simulink model "HIL_Testing_SW"  (Simulink 7.5)
settings: Solver=ode1  StartTime=0.0  StopTime=Inf  FixedStep=0.001  RelTol=1e-3
PostLoadFcn:
  | , if any(exist('dsrtsu_mdlpostloadfcn', 'file') == [2, 3, 6]), try dsrtsu_mdlpostloadfcn('Execute', bdroot); catch fprintf('Error in PostLoadFcn (dsrtsu_mdlpostloadfcn) for model "%s":\n %s\n', bdroot, lasterr); end, end,
undefined symbols (not defined in the file): CeBSER_Cnt_NumTempAxisPts, ChargeCord, ChargeCord_Control, ChargeToSOCCurr, ChrgCurrLim, CrntSens1Fine, CS_SOCSetPt, CyclerMaxChrgPwr, CyclerMaxDschrgPwr, deltaAhr, Drive_1, Drive_10, Drive_11, Drive_12, Drive_13, Drive_14, Drive_15, Drive_16, Drive_17, Drive_18, Drive_19, Drive_2, Drive_20, Drive_21, Drive_22, Drive_23, Drive_24, Drive_25, Drive_26, Drive_27, Drive_28, Drive_29, Drive_3, Drive_30, Drive_31, Drive_32, Drive_33, Drive_34, Drive_35, Drive_36, Drive_37, Drive_38, Drive_39, Drive_4, Drive_40, Drive_41, Drive_42, Drive_43, Drive_44, Drive_45, Drive_46, Drive_47, Drive_48, Drive_49, Drive_5, Drive_50, Drive_51, Drive_6, Drive_7, Drive_8 ... (+50)
libraries: simulink x129, rtican x50, rti2211sailib x5, rti2211serlib x5, rti2202miolib x3
(part 2 of 23)

== system HIL_Testing_SW/HWO ==
  note: 54A Up is down for DIOs
  ChargeMode : Inport  OutDataType=fixdt(1, 16)  OutScaling=2^0
  PackVoltage : Inport  Port=2  OutDataType=fixdt(1, 16)  OutScaling=2^0
  PackCurrent : Inport  Port=3  OutDataType=fixdt(1, 16)  OutScaling=2^0
  Acc : Constant  Value=0  OutDataTypeMode=boolean  OutDataType=sfix(16)  OutScaling=2^0  OutDataTypeStr=boolean
  AccReset : Constant  Value=0  OutDataTypeMode=boolean  OutDataType=sfix(16)  OutScaling=2^0  OutDataTypeStr=boolean
  Charge : Subsystem
  Compare To Zero1 : simulink/Logic and Bit Operations/Compare To Zero  SystemSampleTime=-1  relop===  LogicOutDataTypeMode=uint8  ZeroCross=off
  Constant : Constant  OutDataType=fixdt(1, 16)  OutScaling=2^0
  ContactorLineActive : Constant  OutDataTypeMode=boolean  OutDataType=fixdt(1, 16)  OutScaling=2^0  OutDataTypeStr=boolean
  DS2202BIT_OUT_B2_C1 : rti2202miolib/DS2202BIT_OUT_B1_C1  SystemSampleTime=-1  DSProperties=struct('RTI',struct('Version',uint32(1),'BlockType',struct('isSLSource',uint8(0),'isSLSink',uint8(1),'isHWSource',uint8(0),'isHWSink',uint8(1),'isSetup',uint8(0),'isInline',uint8(1),'isNonInline',uint8(0),'isInterrupt',uint8(0),'isChannelwise',uint8(1)),'IOBoardType',{{'DS2202','MIO'}},'UnitType','BIT','Identifier','BITOUTCH','DialogType','ML','BlockSet','NONE','SlaveProcessor','NONE'))  RTIBlockInterface=struct('InputPortsWidth',int32(1),'InputPortsActive',1,'InputPortsDataType',{{'SS_BOOLEAN'}},'InputPortsName',{{'BITCH_in'}},'BlockDisplay',{{['BIT OUT\n Channelwise'],'center'}},'IconTransparency','off','InitLevel',2,'DialogFcn','gui2202bitoutch','BlockName',struct('Token',{{'DS2202BIT_OUT_B','_C'}},'BlockParam',{{'BoardNo','ChannelNo'}}),'MaskDescription',['Provides bit-wise write access to the digital output.'],'AddBlockVar',{{'Reserved1','edit','[]';'Reserved2','edit','[]';'Reserved3','edit','[]';'Reserved4','edit','[]'}})  RTIBlockParameters=struct('BoardNo',{{2,'ON',[1 16]}},'ChannelNo',{{1,'ON',[1 16]}},'StateInitValue',{{0,'OFF',[0 1]}},'StateTermMode',{{0,'OFF',[0 1]}},'StateTermValue',{{0,'OFF',[0 1]}},'TLCFileName',{{'rti2202outch','OFF',[]}})  RTISFcnParameters=struct('BoardNo','int32','ChannelNo','int32','StateInitValue','int32','StateTermMode','int32','StateTermValue','int32','TLCFileName','char')  RTIBlockParaDefault=struct('BoardNo',1,'ChannelNo',1,'StateInitValue',0,'StateTermMode',0,'StateTermValue',0,'TLCFileName','rti2202outch')
  DS2202BIT_OUT_B2_C2 : rti2202miolib/DS2202BIT_OUT_B1_C1  SystemSampleTime=-1  DSProperties=struct('RTI',struct('Version',uint32(1),'BlockType',struct('isSLSource',uint8(0),'isSLSink',uint8(1),'isHWSource',uint8(0),'isHWSink',uint8(1),'isSetup',uint8(0),'isInline',uint8(1),'isNonInline',uint8(0),'isInterrupt',uint8(0),'isChannelwise',uint8(1)),'IOBoardType',{{'DS2202','MIO'}},'UnitType','BIT','Identifier','BITOUTCH','DialogType','ML','BlockSet','NONE','SlaveProcessor','NONE'))  RTIBlockInterface=struct('InputPortsWidth',int32(1),'InputPortsActive',1,'InputPortsDataType',{{'SS_BOOLEAN'}},'InputPortsName',{{'BITCH_in'}},'BlockDisplay',{{['BIT OUT\n Channelwise'],'center'}},'IconTransparency','off','InitLevel',2,'DialogFcn','gui2202bitoutch','BlockName',struct('Token',{{'DS2202BIT_OUT_B','_C'}},'BlockParam',{{'BoardNo','ChannelNo'}}),'MaskDescription',['Provides bit-wise write access to the digital output.'],'AddBlockVar',{{'Reserved1','edit','[]';'Reserved2','edit','[]';'Reserved3','edit','[]';'Reserved4','edit','[]'}})  RTIBlockParameters=struct('BoardNo',{{2,'ON',[1 16]}},'ChannelNo',{{2,'ON',[1 16]}},'StateInitValue',{{0,'OFF',[0 1]}},'StateTermMode',{{0,'OFF',[0 1]}},'StateTermValue',{{0,'OFF',[0 1]}},'TLCFileName',{{'rti2202outch','OFF',[]}})  RTISFcnParameters=struct('BoardNo','int32','ChannelNo','int32','StateInitValue','int32','StateTermMode','int32','StateTermValue','int32','TLCFileName','char')  RTIBlockParaDefault=struct('BoardNo',1,'ChannelNo',1,'StateInitValue',0,'StateTermMode',0,'StateTermValue',0,'TLCFileName','rti2202outch')
  DS2211BIT_OUT_B2_C10 : rti2211sailib/DS2211BIT_OUT_B1_C1  SystemSampleTime=-1  DSProperties=struct('RTI',struct('Version',uint32(1),'BlockType',struct('isSLSource',uint8(0),'isSLSink',uint8(1),'isHWSource',uint8(0),'isHWSink',uint8(1),'isSetup',uint8(0),'isInline',uint8(1),'isNonInline',uint8(0),'isInterrupt',uint8(0),'isChannelwise',uint8(1)),'IOBoardType',{{'DS2211','SAI'}},'UnitType','BIT','Identifier','BITOUTCH','DialogType','ML','BlockSet','NONE','SlaveProcessor','NONE'))  RTIBlockInterface=struct('InputPortsWidth',int32(1),'InputPortsActive',1,'InputPortsDataType',{{'SS_BOOLEAN'}},'InputPortsName',{{'BITCH_in'}},'BlockDisplay',{{['BIT OUT\n Channelwise'],'center'}},'IconTransparency','off','InitLevel',2,'DialogFcn','gui2211bitoutch','BlockName',struct('Token',{{'DS2211BIT_OUT_B','_C'}},'BlockParam',{{'BoardNo','ChannelNo'}}),'MaskDescription',['Provides bit-wise write access to the digital output.'],'AddBlockVar',{{'Reserved1','edit','[]';'Reserved2','edit','[]';'Reserved3','edit','[]';'Reserved4','edit','[]'}})  RTIBlockParameters=struct('BoardNo',{{2,'ON',[1 16]}},'ChannelNo',{{10,'ON',[1 16]}},'StateInitValue',{{0,'OFF',[0 1]}},'StateTermMode',{{0,'OFF',[0 1]}},'StateTermValue',{{0,'OFF',[0 1]}},'TLCFileName',{{'rti2211outch','OFF',[]}})  RTISFcnParameters=struct('BoardNo','int32','ChannelNo','int32','StateInitValue','int32','StateTermMode','int32','StateTermValue','int32','TLCFileName','char')  RTIBlockParaDefault=struct('BoardNo',1,'ChannelNo',1,'StateInitValue',0,'StateTermMode',0,'StateTermValue',0,'TLCFileName','rti2211outch')
  DS2211BIT_OUT_B2_C5 : rti2211sailib/DS2211BIT_OUT_B1_C1  SystemSampleTime=-1  DSProperties=struct('RTI',struct('Version',uint32(1),'BlockType',struct('isSLSource',uint8(0),'isSLSink',uint8(1),'isHWSource',uint8(0),'isHWSink',uint8(1),'isSetup',uint8(0),'isInline',uint8(1),'isNonInline',uint8(0),'isInterrupt',uint8(0),'isChannelwise',uint8(1)),'IOBoardType',{{'DS2211','SAI'}},'UnitType','BIT','Identifier','BITOUTCH','DialogType','ML','BlockSet','NONE','SlaveProcessor','NONE'))  RTIBlockInterface=struct('InputPortsWidth',int32(1),'InputPortsActive',1,'InputPortsDataType',{{'SS_BOOLEAN'}},'InputPortsName',{{'BITCH_in'}},'BlockDisplay',{{['BIT OUT\n Channelwise'],'center'}},'IconTransparency','off','InitLevel',2,'DialogFcn','gui2211bitoutch','BlockName',struct('Token',{{'DS2211BIT_OUT_B','_C'}},'BlockParam',{{'BoardNo','ChannelNo'}}),'MaskDescription',['Provides bit-wise write access to the digital output.'],'AddBlockVar',{{'Reserved1','edit','[]';'Reserved2','edit','[]';'Reserved3','edit','[]';'Reserved4','edit','[]'}})  RTIBlockParameters=struct('BoardNo',{{2,'ON',[1 16]}},'ChannelNo',{{5,'ON',[1 16]}},'StateInitValue',{{0,'OFF',[0 1]}},'StateTermMode',{{0,'OFF',[0 1]}},'StateTermValue',{{0,'OFF',[0 1]}},'TLCFileName',{{'rti2211outch','OFF',[]}})  RTISFcnParameters=struct('BoardNo','int32','ChannelNo','int32','StateInitValue','int32','StateTermMode','int32','StateTermValue','int32','TLCFileName','char')  RTIBlockParaDefault=struct('BoardNo',1,'ChannelNo',1,'StateInitValue',0,'StateTermMode',0,'StateTermValue',0,'TLCFileName','rti2211outch')
  DS2211PWM_B2_C7 : rti2211sailib/DS2211PWM_B1_C1  SystemSampleTime=-1  Reserved1=[]  Reserved2=[]  Reserved3=[]  Reserved4=[]  DSProperties=struct('RTI',struct('Version',uint32(1),'BlockType',struct('isSLSource',uint8(0),'isSLSink',uint8(1),'isHWSource',uint8(0),'isHWSink',uint8(1),'isSetup',uint8(0),'isInline',uint8(1),'isNonInline',uint8(0),'isInterrupt',uint8(0),'isChannelwise',uint8(1)),'IOBoardType',{{'DS2211','SAI'}},'UnitType','PWM','Identifier','PWM','DialogType','ML','BlockSet','NONE','SlaveProcessor','NONE'))  RTIBlockInterface=struct('InputPortsWidth',int32([1 1]),'InputPortsActive',[1 1],'InputPortsName',{{['Duty Cycle'],'Period'}},'IconTransparency','on','InitLevel',2,'DialogFcn','gui2211pwm','BlockName',struct('Token',{{'DS2211PWM_B','_C'}},'BlockParam',{{'BoardNo','ChannelNo'}}),'MaskDescription',['Generation of a square-wave-type signal for a given period and duty cycle.'])  RTIBlockParameters=struct('BoardNo',{{2,'ON',[1 16]}},'ChannelNo',{{7,'ON',[1 9]}},'UpdateMode',{{1,'ON',[1 2]}},'PeriodRange',{{2,'OFF',[1 16]}},'DutyCycleInitValue',{{'0.2','OFF',[0 1]}},'PeriodInitValue',{{'1e-005','OFF',[]}},'DutyCyclePeriodTermMode',{{0,'OFF',[0 1]}},'DutyCycleTermValue',{{'0','OFF',[0 1]}},'PeriodTermValue',{{'5e-005','OFF',[]}},'TLCFileName',{{'rti2211pwm','OFF',[]}})  RTISFcnParameters=struct('BoardNo','int32','ChannelNo','int32','UpdateMode','int32','PeriodRange','int32','DutyCycleInitValue','double','PeriodInitValue','double','DutyCyclePeriodTermMode','int32','DutyCycleTermValue','double','PeriodTermValue','double','TLCFileName','char')  RTIBlockParaDefault=struct('BoardNo',1,'ChannelNo',1,'UpdateMode',1,'PeriodRange',7,'DutyCycleInitValue',0,'PeriodInitValue',5e-05,'DutyCyclePeriodTermMode',0,'DutyCycleTermValue',0,'PeriodTermValue',5e-05,'TLCFileName','rti2211pwm')
  DS2211PWM_B2_C9 : rti2211sailib/DS2211PWM_B1_C1  SystemSampleTime=-1  Reserved1=[]  Reserved2=[]  Reserved3=[]  Reserved4=[]  DSProperties=struct('RTI',struct('Version',uint32(1),'BlockType',struct('isSLSource',uint8(0),'isSLSink',uint8(1),'isHWSource',uint8(0),'isHWSink',uint8(1),'isSetup',uint8(0),'isInline',uint8(1),'isNonInline',uint8(0),'isInterrupt',uint8(0),'isChannelwise',uint8(1)),'IOBoardType',{{'DS2211','SAI'}},'UnitType','PWM','Identifier','PWM','DialogType','ML','BlockSet','NONE','SlaveProcessor','NONE'))  RTIBlockInterface=struct('InputPortsWidth',int32([1 1]),'InputPortsActive',[1 1],'InputPortsName',{{['Duty Cycle'],'Period'}},'IconTransparency','on','InitLevel',2,'DialogFcn','gui2211pwm','BlockName',struct('Token',{{'DS2211PWM_B','_C'}},'BlockParam',{{'BoardNo','ChannelNo'}}),'MaskDescription',['Generation of a square-wave-type signal for a given period and duty cycle.'])  RTIBlockParameters=struct('BoardNo',{{2,'ON',[1 16]}},'ChannelNo',{{9,'ON',[1 9]}},'UpdateMode',{{1,'ON',[1 2]}},'PeriodRange',{{3,'OFF',[1 16]}},'DutyCycleInitValue',{{'0.2','OFF',[0 1]}},'PeriodInitValue',{{'1e-005','OFF',[]}},'DutyCyclePeriodTermMode',{{0,'OFF',[0 1]}},'DutyCycleTermValue',{{'0','OFF',[0 1]}},'PeriodTermValue',{{'5e-005','OFF',[]}},'TLCFileName',{{'rti2211pwm','OFF',[]}})  RTISFcnParameters=struct('BoardNo','int32','ChannelNo','int32','UpdateMode','int32','PeriodRange','int32','DutyCycleInitValue','double','PeriodInitValue','double','DutyCyclePeriodTermMode','int32','DutyCycleTermValue','double','PeriodTermValue','double','TLCFileName','char')  RTIBlockParaDefault=struct('BoardNo',1,'ChannelNo',1,'UpdateMode',1,'PeriodRange',7,'DutyCycleInitValue',0,'PeriodInitValue',5e-05,'DutyCyclePeriodTermMode',0,'DutyCycleTermValue',0,'PeriodTermValue',5e-05,'TLCFileName','rti2211pwm')
  Data Store Read : DataStoreRead  DataStoreName=fault  SampleTime=0
  Data Store Read1 : DataStoreRead  DataStoreName=ResetRun  SampleTime=0
  Data Store Read2 : DataStoreRead  DataStoreName=ResetRun  SampleTime=0
  Data Store Write : DataStoreWrite  DataStoreName=ContactorLine  SampleTime=-1
  Data Store Write1 : DataStoreWrite  DataStoreName=ACC  SampleTime=-1
  Data Store Write2 : DataStoreWrite  DataStoreName=RUN  SampleTime=-1
  Divide : Product  Inputs=*/  OutDataType=fixdt(1, 16)  OutScaling=2^-10
  DriveSelect4 : Switch  Threshold=0.5  OutDataType=fixdt(1, 16)  OutScaling=2^0
  DriveSelect6 : Switch  Threshold=0.5  OutDataType=fixdt(1, 16)  OutScaling=2^0
  Logical Operator : Logic  Operator=NOT  AllPortsSameDT=off  OutDataTypeMode=boolean  LogicDataType=fixdt(0, 8)  OutDataTypeStr=boolean
  Logical Operator3 : Logic  AllPortsSameDT=off  OutDataTypeMode=boolean  LogicDataType=fixdt(0, 8)  OutDataTypeStr=boolean
  Logical Operator8 : Logic  Operator=OR  AllPortsSameDT=off  OutDataTypeMode=boolean  LogicDataType=fixdt(0, 8)  OutDataTypeStr=boolean
  Reset_Run : Constant  Value=0  OutDataTypeMode=boolean  OutDataType=fixdt(1, 16)  OutScaling=2^0  OutDataTypeStr=boolean
  Run : Constant  Value=0  OutDataTypeMode=boolean  OutDataType=fixdt(1, 16)  OutScaling=2^0  OutDataTypeStr=boolean
  Switch1 : Switch  Threshold=.5  OutDataType=fixdt(1, 16)  OutScaling=2^0
  TX HVEM : Subsystem
  Ignition : Outport  OutDataType=fixdt(1, 16)  OutScaling=2^0
  tag scope: ChargeMode=global, Ignition=global, PackCurrent=global, PackVoltage=global
  wires:
  [DC] -> DS2211PWM_B2_C7/1
  [Period] -> DS2211PWM_B2_C7/2
  [Prox] -> DS2211BIT_OUT_B2_C5/1
  AccReset/1 -> DriveSelect6/1
  Data Store Read2/1 -> DriveSelect6/2
  DriveSelect6/1 -> Data Store Write1/1, DS2202BIT_OUT_B2_C1/1
  DriveSelect4/1 -> DS2211BIT_OUT_B2_C10/1, Data Store Write/1
  ContactorLineActive/1 -> DriveSelect4/1
  [ChargeMode] -> DriveSelect4/2
  [Ignition] -> Logical Operator3/1
  Data Store Read/1 -> Compare To Zero1/1
  Compare To Zero1/1 -> Logical Operator3/2
  Logical Operator3/1 -> DriveSelect4/3
  Acc/1 -> DriveSelect6/3
  Switch1/1 -> Ignition/1, Data Store Write2/1, [Ignition], DS2202BIT_OUT_B2_C2/1
  Reset_Run/1 -> Switch1/1
  Run/1 -> Switch1/3
  Logical Operator8/1 -> Switch1/2
  Data Store Read1/1 -> Logical Operator8/1
  ChargeMode/1 -> [ChargeMode]
  [ChargeMode] -> Logical Operator8/2
  Logical Operator/1 -> Charge/Enable
  [ChargeMode] -> Logical Operator/1
  Charge/1(Period_1) -> [Period1]
  Charge/2(DC1) -> [DC1]
  Charge/3(Prox) -> [Prox1]
  TX HVEM/1(DC) -> [DC]
  TX HVEM/2(Period) -> [Period]
  TX HVEM/3(Proximity) -> [Prox]
  [PackCurrent] -> TX HVEM/1(Current)
  [ChargeMode] -> TX HVEM/2(CM)
  [PackVoltage] -> TX HVEM/3(Voltage)
  PackVoltage/1 -> [PackVoltage]
  PackCurrent/1 -> [PackCurrent]
  TX HVEM/4(PrcsdVolt_DC) -> [PrcsdVolt_DC]
  TX HVEM/5(PrcsdVolt_Period) -> [PrcsdVolt_Freq]
  [PrcsdVolt_Freq] -> DS2211PWM_B2_C9/2
  Constant/1 -> Divide/2
  [PrcsdVolt_DC] -> Divide/1
  Divide/1 -> DS2211PWM_B2_C9/1

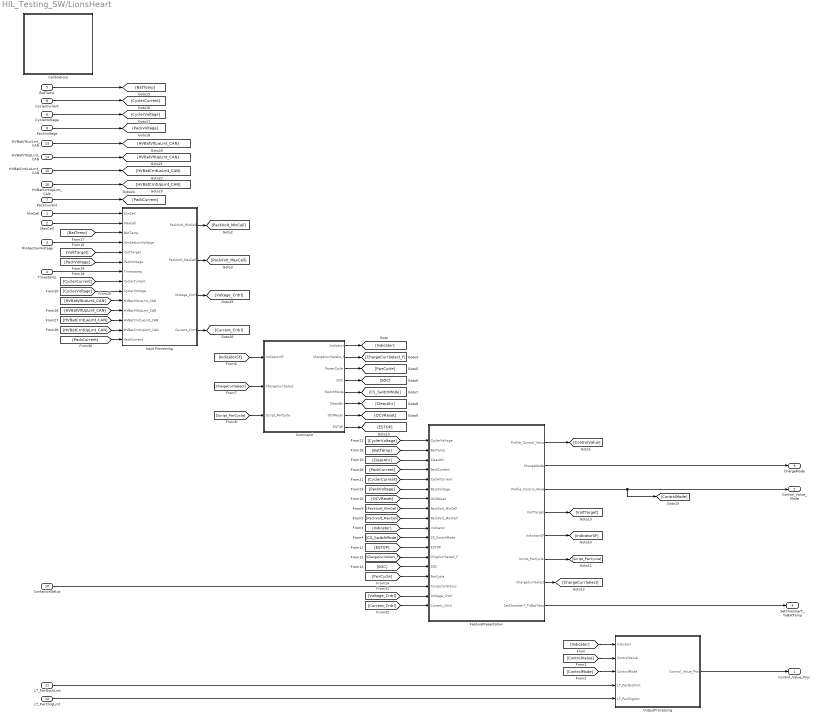
== system HIL_Testing_SW/LionsHeart ==
  MinCell : Inport  OutDataType=fixdt(1, 16)  OutScaling=2^0
  MaxCell : Inport  Port=2  OutDataType=fixdt(1, 16)  OutScaling=2^0
  MinSectionVoltage : Inport  Port=3  OutDataType=fixdt(1, 16)  OutScaling=2^0
  Timestamp : Inport  Port=4  OutDataType=fixdt(1, 16)  OutScaling=2^0
  BatTemp : Inport  Port=5  OutDataType=fixdt(1, 16)  OutScaling=2^0
  CyclerVoltage : Inport  Port=6  OutDataType=fixdt(1, 16)  OutScaling=2^0
  PackCurrent : Inport  Port=7  OutDataType=fixdt(1, 16)  OutScaling=2^0
  CyclerCurrent : Inport  Port=8  OutDataType=fixdt(1, 16)  OutScaling=2^0
  PackVoltage : Inport  Port=9  OutDataType=fixdt(1, 16)  OutScaling=2^0
  ContactorStatus : Inport  Port=10  OutDataType=fixdt(1, 16)  OutScaling=2^0
  LT_PwrDschLmt : Inport  Port=11  OutDataType=fixdt(1, 16)  OutScaling=2^0
  LT_PwrChrgLmt : Inport  Port=12  OutDataType=fixdt(1, 16)  OutScaling=2^0
  HVBatVltLwLmt_CAN : Inport  Port=13  OutDataType=fixdt(1, 16)  OutScaling=2^0
  HVBatVltUpLmt_CAN : Inport  Port=14  OutDataType=fixdt(1, 16)  OutScaling=2^0
  HVBatCrntLwLmt_CAN : Inport  Port=15  OutDataType=fixdt(1, 16)  OutScaling=2^0
  HVBatCrntUpLmt_CAN : Inport  Port=16  OutDataType=fixdt(1, 16)  OutScaling=2^0
  Calibrations : Subsystem
  Command : Subsystem
  FeaturePresentation : Subsystem
  Input Processing : Subsystem
  OutputProcessing : Subsystem
  Control_Value_Proc : Outport  OutDataType=fixdt(1, 16)  OutScaling=2^0
  Control_Value_Mode : Outport  Port=2  OutDataType=fixdt(1, 16)  OutScaling=2^0
  ChargeMode : Outport  Port=3  OutDataType=fixdt(1, 16)  OutScaling=2^0
  SetChamberT_ToBatTemp : Outport  Port=4  OutDataType=fixdt(1, 16)  OutScaling=2^0
  wires:
  OutputProcessing/1(Control_Value_Proc) -> Control_Value_Proc/1
  LT_PwrDschLmt/1 -> OutputProcessing/4(LT_PwrDschlmt)
  LT_PwrChrgLmt/1 -> OutputProcessing/5(LT_PwrChgLmt)
  Command/1(Indicator) -> [Indicator]
  [Indicator] -> OutputProcessing/1(Indicator)
  FeaturePresentation/1(Profile_Control_Value) -> [ControlValue]
  FeaturePresentation/3(Profile_Control_Mode) -> Control_Value_Mode/1, [ControlMode]
  [ControlValue] -> OutputProcessing/2(ControlValue)
  [ControlMode] -> OutputProcessing/3(ControlMode)
  [Indicator] -> FeaturePresentation/10(Indicator)
  Input Processing/1(PackVolt_MinCell) -> [PackVolt_MinCell]
  Input Processing/2(PackVolt_MaxCell) -> [PackVolt_MaxCell]
  FeaturePresentation/2(ChargeMode) -> ChargeMode/1
  [CS_SwitchMode] -> FeaturePresentation/11(CS_SwitchMode)
  [PackVolt_MaxCell] -> FeaturePresentation/9(PackVolt_MaxCell)
  Command/2(ChargeCurrSelect_F) -> [ChargeCurrSelect_F]
  Command/3(PowerCycle) -> [PwrCycle]
  Command/4(SOC) -> [SOC]
  Command/5(SwitchMode) -> [CS_SwitchMode]
  Command/6(ClearAhr) -> [ClearAhr]
  Command/7(OCVReset) -> [OCVReset]
  [IndicatorSF] -> Command/1(IndicatorSF)
  [ChargeCurrSelect] -> Command/2(ChargeCurrSelect)
  FeaturePresentation/5(IndicatorSF) -> [IndicatorSF]
  FeaturePresentation/6(Script_PwrCycle) -> [Script_PwrCycle]
  FeaturePresentation/7(ChargeCurrSelect) -> [ChargeCurrSelect]
  FeaturePresentation/4(VoltTarget) -> [VoltTarget]
  [Script_PwrCycle] -> Command/3(Script_PwrCycle)
  [PackVolt_MinCell] -> FeaturePresentation/8(PackVolt_MinCell)
  [OCVReset] -> FeaturePresentation/7(OCVReset)
  Command/8(ESTOP) -> [ESTOP]
  [ESTOP] -> FeaturePresentation/12(ESTOP)
  [ChargeCurrSelect_F] -> FeaturePresentation/13(ChrgCurrSelect_F)
  [SOC] -> FeaturePresentation/14(SOC)
  [PwrCycle] -> FeaturePresentation/15(PwrCycle)
  [ClearAhr] -> FeaturePresentation/3(ClearAhr)
  [VoltTarget] -> Input Processing/5(VoltTarget)
  MinCell/1 -> Input Processing/1(MinCell)
  MaxCell/1 -> Input Processing/2(MaxCell)
  MinSectionVoltage/1 -> Input Processing/4(MinSectionVoltage)
  Timestamp/1 -> Input Processing/7(Timestamp)
  BatTemp/1 -> [BatTemp]
  [BatTemp] -> Input Processing/3(BatTemp)
  [BatTemp] -> FeaturePresentation/2(BatTemp)
  ContactorStatus/1 -> FeaturePresentation/16(ContactorStatus)
  CyclerCurrent/1 -> [CyclerCurrent]
  CyclerVoltage/1 -> [CyclerVoltage]
  [CyclerCurrent] -> Input Processing/8(CyclerCurrent)
  [CyclerVoltage] -> Input Processing/9(CyclerVotlage)
  [CyclerCurrent] -> FeaturePresentation/5(CyclerCurrent)
  [CyclerVoltage] -> FeaturePresentation/1(CyclerVoltage)
  [PackVoltage] -> FeaturePresentation/6(PackVoltage)
  PackVoltage/1 -> [PackVoltage]
  [PackVoltage] -> Input Processing/6(PackVoltage)
  HVBatVltLwLmt_CAN/1 -> [HVBatVltLwLmt_CAN]
  HVBatVltUpLmt_CAN/1 -> [HVBatVltUpLmt_CAN]
  HVBatCrntLwLmt_CAN/1 -> [HVBatCrntLwLmt_CAN]
  HVBatCrntUpLmt_CAN/1 -> [HVBatCrntUpLmt_CAN]
  [HVBatVltLwLmt_CAN] -> Input Processing/10(HVBatVltLwLmt_CAN)
  [HVBatVltUpLmt_CAN] -> Input Processing/11(HVBatVltUpLmt_CAN)
  [HVBatCrntLwLmt_CAN] -> Input Processing/12(HVBatCrntLwLmt_CAN)
  [HVBatCrntUpLmt_CAN] -> Input Processing/13(HVBatCrntUpLmt_CAN)
  PackCurrent/1 -> [PackCurrent]
  [PackCurrent] -> FeaturePresentation/4(PackCurrent)
  [PackCurrent] -> Input Processing/14(PackCurrent)
  Input Processing/3(Voltage_Cntrl) -> [Voltage_Cntrl]
  Input Processing/4(Current_Cntrl) -> [Current_Cntrl]
  [Voltage_Cntrl] -> FeaturePresentation/17(Voltage_Cntrl)
  [Current_Cntrl] -> FeaturePresentation/18(Current_Cntrl)
  FeaturePresentation/8(SetChamberT_ToBatTemp) -> SetChamberT_ToBatTemp/1

== system HIL_Testing_SW/RTI Data ==
  RTI Data Store : Subsystem  Tag="struct('private',struct('version',struct('dsVer',uint32(2),'dsVerCreation',uint32(2),'RTI',struct('ver','6.7','type','RTI1006')),'access',struct('type','Model','isPerm',1,'created',['10-Dec-2012 12:09:16'],'modified',['22-Sep-2015 13:45:03'],'location','')),'public',struct('main',struct('data',[]),'sub',struct('name',{{'HIL_Testing_SW'}},'data',{{struct('TH',struct('thTaskInfo',struct('taskType',{'TIMER','HWINT','TMRINT','SWINT'},'tasksNumOf',{7,0,0,0},'srcIds',{{'TIMERA','TIMERA2','TIMERA3','TIMERA4','TIMERA5','TIMERA6','TIMERA7'},{},{},{}},'taskNames',{{['Timer Task 1'],['Timer Task 2'],['Timer Task 3'],['Timer Task 4'],['Timer Task 5'],['Timer Task 6'],['Timer Task 7']},{},{},{}})),'th_tc',struct('dataType',{'TASK','TASK','TASK','TASK','TASK','TASK','TASK'},'taskGroupId',{'','','','','','',''},'taskGroupList',{{},{},{},{},{},{},{}},'taskSchedulingPolicy',{'FCFS','FCFS','FCFS','FCFS','FCFS','FCFS','FCFS'},'taskType',{'TIMER','TIMER','TIMER','TIMER','TIMER','TIMER','TIMER'},'blkh',{-1,-1,-1,-1,-1,-1,-1},'srcId',{'TIMERA','TIMERA2','TIMERA3','TIMERA4','TIMERA5','TIMERA6','TIMERA7'},'srcSgnName',{['Timer A interrupt'],['Timer Task 1'],['Timer Task 1'],['Timer Task 1'],['Timer Task 1'],['Timer Task 1'],['Timer Task 1']},'srcCpuName',{'','','','','','',''},'taskName',{['Timer Task 1  [0.001] s'],['Timer Task 2  [0.012] s'],['Timer Task 3  [0.025] s'],['Timer Task 4  [0.2] s'],['Timer Task 5  [0.3] s'],['Timer Task 6  [0.4] s'],['Timer Task 7  [1] s']},'taskNameDisplayExt',{'','','','','','',''},'smplTime',{0.001,0.012,0.025,0.2,0.3,0.4,1},'smplTimeOffs',{0,0,0,0,0,0,0},'hasFixedPriority',{0,0,0,0,0,0,0},'priority',{1,2,3,4,5,6,7},'hasFixedOvc',{0,0,0,0,0,0,0},'ovcType',{1,1,1,1,1,1,1},'ovcMax',{1,1,1,1,1,1,1}),'tc_th',struct('dataType',{'TASK','TASK','TASK','TASK','TASK','TASK','TASK'},'taskGroupId',{'','','','','','',''},'taskGroupList',{{},{},{},{},{},{},{}},'taskSchedulingPolicy',{'FCFS','FCFS','FCFS','FCFS','FCFS','FCFS','FCFS'},'taskType',{'TIMER','TIMER','TIMER','TIMER','TIMER','TIMER','TIMER'},'blkh',{-1,-1,-1,-1,-1,-1,-1},'srcId',{'TIMERA','TIMERA2','TIMERA3','TIMERA4','TIMERA5','TIMERA6','TIMERA7'},'srcSgnName',{['Timer A interrupt'],['Timer Task 1'],['Timer Task 1'],['Timer Task 1'],['Timer Task 1'],['Timer Task 1'],['Timer Task 1']},'srcCpuName',{'','','','','','',''},'taskName',{['Timer Task 1  [0.001] s'],['Timer Task 2  [0.012] s'],['Timer Task 3  [0.025] s'],['Timer Task 4  [0.2] s'],['Timer Task 5  [0.3] s'],['Timer Task 6  [0.4] s'],['Timer Task 7  [1] s']},'taskNameDisplayExt',{'','','','','','',''},'smplTime',{0.001,0.012,0.025,0.2,0.3,0.4,1},'smplTimeOffs',{0,0,0,0,0,0,0},'hasFixedPriority',{0,0,0,0,0,0,0},'priority',{1,2,3,4,5,6,7},'hasFixedOvc',{0,0,0,0,0,0,0},'ovcType',{1,1,1,1,1,1,1},'ovcMax',{1,1,1,1,1,1,1}))}})))"
      mask Type: RTI_DATA_STORE
      mask Description:
      | RTI Data Store Block. This block is used by RTI to store internal model dependent data. Deleting this block will result in data loss.
      | 
      | NEVER DELETE, COPY, OR MODIFY THIS BLOCK!
      mask Help:
      | RTI Data Store Block. This block is used by RTI to store internal model dependent data. Deleting this block will result in data loss.
      | 
      | NEVER DELETE, COPY, OR MODIFY THIS BLOCK!
      mask Display: text(0.5, 0.5, ' ', 'HorizontalAlignment', 'center');

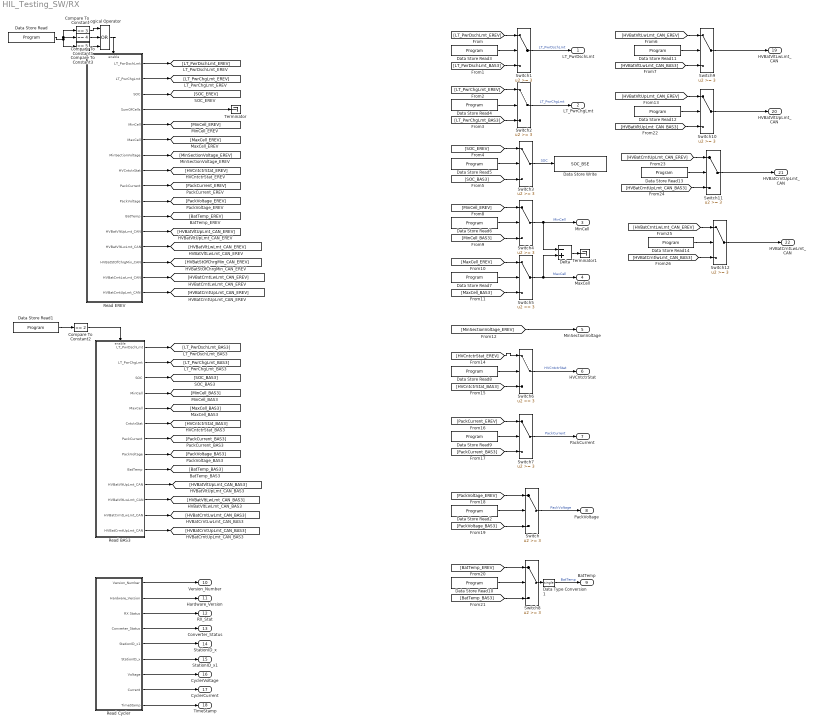
== system HIL_Testing_SW/RX ==
  Compare To Constant : simulink/Logic and Bit Operations/Compare To Constant  SystemSampleTime=-1  relop===  const=3  LogicOutDataTypeMode=uint8
  Compare To Constant1 : simulink/Logic and Bit Operations/Compare To Constant  SystemSampleTime=-1  relop===  const=4  LogicOutDataTypeMode=uint8
  Compare To Constant2 : simulink/Logic and Bit Operations/Compare To Constant  SystemSampleTime=-1  relop===  const=2  LogicOutDataTypeMode=uint8
  Compare To Constant3 : simulink/Logic and Bit Operations/Compare To Constant  SystemSampleTime=-1  relop===  const=5  LogicOutDataTypeMode=uint8
  Data Store Read{,1..14} (15 alike) : DataStoreRead  DataStoreName=Program  SampleTime=0
  Data Store Write : DataStoreWrite  DataStoreName=SOC_BSE  SampleTime=-1
  Data Type Conversion1 : DataTypeConversion  OutDataTypeMode=single  OutDataType=fixdt(1, 16)  OutScaling=2^0  OutDataTypeStr=single
  Delta : Sum  Inputs=-+  OutDataType=fixdt(1, 16)  OutScaling=2^-10
  Logical Operator : Logic  Operator=OR  Inputs=3  AllPortsSameDT=off  OutDataTypeMode=boolean  LogicDataType=fixdt(0, 8)  OutDataTypeStr=boolean
  Read BAS3 : Subsystem
  Read Cycler : Subsystem
  Read EREV : Subsystem
  Switch{,1..12} (13 alike) : Switch  Threshold=3  OutDataType=sfix(16)  OutScaling=2^0
  Terminator : Terminator
  Terminator1 : Terminator
  LT_PwrDschLmt : Outport  OutDataType=fixdt(1, 16)  OutScaling=2^0
  LT_PwrChgLmt : Outport  Port=2  OutDataType=fixdt(1, 16)  OutScaling=2^0
  MinCell : Outport  Port=3  OutDataType=fixdt(1, 16)  OutScaling=2^0
  MaxCell : Outport  Port=4  OutDataType=fixdt(1, 16)  OutScaling=2^0
  MinSectionVoltage : Outport  Port=5  OutDataType=fixdt(1, 16)  OutScaling=2^0
  HVCntctrStat : Outport  Port=6  OutDataType=fixdt(1, 16)  OutScaling=2^0
  PackCurrent : Outport  Port=7  OutDataType=fixdt(1, 16)  OutScaling=2^0
  PackVoltage : Outport  Port=8  OutDataType=fixdt(1, 16)  OutScaling=2^0
  BatTemp : Outport  Port=9  OutDataType=fixdt(1, 16)  OutScaling=2^0
  Version_Number : Outport  Port=10  OutDataType=fixdt(1, 16)  OutScaling=2^0
  Hardware_Version : Outport  Port=11  OutDataType=fixdt(1, 16)  OutScaling=2^0
  RX_Stat : Outport  Port=12  OutDataType=fixdt(1, 16)  OutScaling=2^0
  Converter_Status : Outport  Port=13  OutDataType=fixdt(1, 16)  OutScaling=2^0
  StationID_x : Outport  Port=14  OutDataType=fixdt(1, 16)  OutScaling=2^0
  StationID_x1 : Outport  Port=15  OutDataType=fixdt(1, 16)  OutScaling=2^0
  CyclerVoltage : Outport  Port=16  OutDataType=fixdt(1, 16)  OutScaling=2^0
  CyclerCurrent : Outport  Port=17  OutDataType=fixdt(1, 16)  OutScaling=2^0
  TimeStamp : Outport  Port=18  OutDataType=fixdt(1, 16)  OutScaling=2^0
  HVBatVltLwLmt_CAN : Outport  Port=19  OutDataType=fixdt(1, 16)  OutScaling=2^0
  HVBatVltUpLmt_CAN : Outport  Port=20  OutDataType=fixdt(1, 16)  OutScaling=2^0
  HVBatCrntUpLmt_CAN : Outport  Port=21  OutDataType=fixdt(1, 16)  OutScaling=2^0
  HVBatCrntLwLmt_CAN : Outport  Port=22  OutDataType=fixdt(1, 16)  OutScaling=2^0
  wires:
  Read EREV/2(LT_PwrChgLmt) -> [LT_PwrChgLmt_EREV]
  Read EREV/1(LT_PwrDschLmt) -> [LT_PwrDschLmt_EREV]
  Read EREV/3(SOC) -> [SOC_EREV]
  Read EREV/4(SumOfCells) -> Terminator/1
  Read EREV/5(MinCell) -> [MinCell_EREV]
  Read EREV/6(MaxCell) -> [MaxCell_EREV]
  Read EREV/7(MinSectionVoltage) -> [MinSectionVoltage_EREV]
  Read EREV/8(HVCntctrStat) -> [HVCntctrStat_EREV]
  Read EREV/9(PackCurrent) -> [PackCurrent_EREV]
  Read EREV/10(PackVoltage) -> [PackVoltage_EREV]
  Read EREV/11(BatTemp) -> [BatTemp_EREV]
  Switch/1 -> PackVoltage/1  "PackVoltage"
  Read BAS3/1(LT_PwrDschLmt) -> [LT_PwrDschLmt_BAS3]
  Read BAS3/2(LT_PwrChgLmt) -> [LT_PwrChgLmt_BAS3]
  Read BAS3/3(SOC) -> [SOC_BAS3]
  Read BAS3/4(MinCell) -> [MinCell_BAS3]
  Read BAS3/5(MaxCell) -> [MaxCell_BAS3]
  Read BAS3/6(CntctrStat) -> [HVCntctrStat_BAS3]
  Read BAS3/7(PackCurrent) -> [PackCurrent_BAS3]
  Read BAS3/8(PackVoltage) -> [PackVoltage_BAS3]
  Read BAS3/9(BatTemp) -> [BatTemp_BAS3]
  [MinSectionVoltage_EREV] -> MinSectionVoltage/1
  Data Store Read/1 -> Compare To Constant/1, Compare To Constant1/1, Compare To Constant3/1
  Compare To Constant/1 -> Logical Operator/1
  Compare To Constant1/1 -> Logical Operator/2
  Logical Operator/1 -> Read EREV/Enable
  Data Store Read1/1 -> Compare To Constant2/1
  Compare To Constant2/1 -> Read BAS3/Enable
  Read Cycler/1(Version_Number) -> Version_Number/1
  Read Cycler/2(Hardware_Version) -> Hardware_Version/1
  Read Cycler/3(RX Status) -> RX_Stat/1
  Read Cycler/4(Converter_Status) -> Converter_Status/1
  Read Cycler/5(StationID_x1) -> StationID_x/1
  Read Cycler/6(StationID_x) -> StationID_x1/1
  Read Cycler/7(Voltage) -> CyclerVoltage/1
  Read Cycler/8(Current) -> CyclerCurrent/1
  Read Cycler/9(TimeStamp) -> TimeStamp/1
  Data Type Conversion1/1 -> BatTemp/1  "BatTemp"
  Data Store Read2/1 -> Switch/2
  [PackVoltage_BAS3] -> Switch/3
  [PackVoltage_EREV] -> Switch/1
  [LT_PwrDschLmt_BAS3] -> Switch1/3
  [LT_PwrDschLmt_EREV] -> Switch1/1
  Data Store Read3/1 -> Switch1/2
  Switch1/1 -> LT_PwrDschLmt/1  "LT_PwrDschLmt"
  Data Store Read4/1 -> Switch2/2
  [LT_PwrChgLmt_EREV] -> Switch2/1
  [LT_PwrChgLmt_BAS3] -> Switch2/3
  Switch2/1 -> LT_PwrChgLmt/1  "LT_PwrChgLmt"
  [SOC_EREV] -> Switch3/1
  [SOC_BAS3] -> Switch3/3
  Data Store Read5/1 -> Switch3/2
  Switch3/1 -> Data Store Write/1  "SOC"
  [MinCell_BAS3] -> Switch4/3
  [MinCell_EREV] -> Switch4/1
  Data Store Read6/1 -> Switch4/2
  Switch4/1 -> MinCell/1, Delta/1  "MinCell"
  [MaxCell_EREV] -> Switch5/1
  [MaxCell_BAS3] -> Switch5/3
  Data Store Read7/1 -> Switch5/2
  Switch5/1 -> MaxCell/1, Delta/2  "MaxCell"
  [HVCntctrStat_EREV] -> Switch6/1
  [HVCntctrStat_BAS3] -> Switch6/3
  Data Store Read8/1 -> Switch6/2
  Switch6/1 -> HVCntctrStat/1  "HVCntctrStat"
  [PackCurrent_EREV] -> Switch7/1
  [PackCurrent_BAS3] -> Switch7/3
  Data Store Read9/1 -> Switch7/2
  Switch7/1 -> PackCurrent/1  "PackCurrent"
  [BatTemp_EREV] -> Switch8/1
  [BatTemp_BAS3] -> Switch8/3
  Data Store Read10/1 -> Switch8/2
  Switch8/1 -> Data Type Conversion1/1
  Read EREV/12(HVBatVltUpLmt_CAN) -> [HVBatVltUpLmt_CAN_EREV]
  Read EREV/13(HVBatVltLwLmt_CAN) -> [HVBatVltLwLmt_CAN_EREV]
  Read EREV/14(HVBatStOfChrgMin_CAN) -> [HVBatStOfChrgMin_CAN_EREV]
  Read EREV/15(HVBatCrntLwLmt_CAN) -> [HVBatCrntLwLmt_CAN_EREV]
  Read EREV/16(HVBatCrntUpLmt_CAN) -> [HVBatCrntUpLmt_CAN_EREV]
  Read BAS3/10(HVBatVltUpLmt_CAN) -> [HVBatVltUpLmt_CAN_BAS3]
  [HVBatVltLwLmt_CAN_BAS3] -> Switch9/3
  [HVBatVltLwLmt_CAN_EREV] -> Switch9/1
  Data Store Read11/1 -> Switch9/2
  Read BAS3/11(HVBatVltLwLmt_CAN) -> [HVBatVltLwLmt_CAN_BAS3]
  Read BAS3/12(HVBatCrmtLwLmt_CAN) -> [HVBatCrntLwLmt_CAN_BAS3]
  Read BAS3/13(HVBatCrmtUpLmt_CAN) -> [HVBatCrntUpLmt_CAN_BAS3]
  Switch9/1 -> HVBatVltLwLmt_CAN/1
  [HVBatVltUpLmt_CAN_BAS3] -> Switch10/3
  [HVBatVltUpLmt_CAN_EREV] -> Switch10/1
  Data Store Read12/1 -> Switch10/2
  Switch10/1 -> HVBatVltUpLmt_CAN/1
  [HVBatCrntUpLmt_CAN_BAS3] -> Switch11/3
  [HVBatCrntUpLmt_CAN_EREV] -> Switch11/1
  Data Store Read13/1 -> Switch11/2
  Switch11/1 -> HVBatCrntUpLmt_CAN/1
  [HVBatCrntlwLmt_CAN_BAS3] -> Switch12/3
  [HVBatCrntLwLmt_CAN_EREV] -> Switch12/1
  Data Store Read14/1 -> Switch12/2
  Switch12/1 -> HVBatCrntLwLmt_CAN/1
  Compare To Constant3/1 -> Logical Operator/3
  Delta/1 -> Terminator1/1

== system HIL_Testing_SW/TX ==
  note: Place holder for future use!
      | SDE 0821
  Version_Number : Inport  OutDataType=sfix(16)  OutScaling=2^0
  Hardware_Version : Inport  Port=2  OutDataType=sfix(16)  OutScaling=2^0
  Rx_status : Inport  Port=3  OutDataType=sfix(16)  OutScaling=2^0
  Converter_Status : Inport  Port=4  OutDataType=sfix(16)  OutScaling=2^0
  StationID_x1 : Inport  Port=5  OutDataType=sfix(16)  OutScaling=2^0
  StationID_x : Inport  Port=6  OutDataType=sfix(16)  OutScaling=2^0
  Control_Value_Proc : Inport  Port=7  OutDataType=sfix(16)  OutScaling=2^0
  Control_Mode : Inport  Port=8  OutDataType=sfix(16)  OutScaling=2^0
  BatTemp : Inport  Port=9  OutDataType=sfix(16)  OutScaling=2^0
  PackVoltage : Inport  Port=10  OutDataType=sfix(16)  OutScaling=2^0
  Ignition : Inport  Port=11  OutDataType=sfix(16)  OutScaling=2^0
  SetChamberT_ToBatTemp : Inport  Port=12  OutDataType=sfix(16)  OutScaling=2^0
  Chamber : Subsystem
  Chiller : Subsystem
  Data Store Read : DataStoreRead  DataStoreName=ContactorLine  SampleTime=0
  Data Store Read1 : DataStoreRead  DataStoreName=ContactorLine  SampleTime=0
  Data Store Read2 : DataStoreRead  DataStoreName=ContactorLine  SampleTime=0
  ProfBatt_Temp : Constant  Value=single(25.1)  OutDataType=fixdt(1, 16)  OutScaling=2^0
  PrpslnAtv : Subsystem
  TX PTEI : Subsystem
  Tx_Cycler : Subsystem
  wires:
  Version_Number/1 -> Tx_Cycler/3(Version_Number)
  Hardware_Version/1 -> Tx_Cycler/4(Hardware_Version)
  Rx_status/1 -> Tx_Cycler/5(Rx_status)
  Converter_Status/1 -> Tx_Cycler/6(Converter_Status_B)
  Data Store Read1/1 -> TX PTEI/3(ContactorLine)
  Data Store Read2/1 -> PrpslnAtv/1(ContactorLine)
  BatTemp/1 -> [Temp]
  PackVoltage/1 -> [PackVoltage]
  Ignition/1 -> [Ignition]
  [PackVoltage] -> TX PTEI/1(BatVolt)
  [Ignition] -> TX PTEI/2(Ignition)
  Control_Value_Proc/1 -> Tx_Cycler/1(Control_Value_Proc)
  Control_Mode/1 -> Tx_Cycler/2(Control_Mode)
  StationID_x1/1 -> Tx_Cycler/7(StationID_B1)
  StationID_x/1 -> Tx_Cycler/8(StationID_B)
  [Temp] -> Chamber/1(BatTemp)
  SetChamberT_ToBatTemp/1 -> [SetChamberT_ToBatTemp]
  [SetChamberT_ToBatTemp] -> Chamber/2(SetChamberT_ToBatTemp)
  [Temp] -> Chiller/1(BatTemp)
  Data Store Read/1 -> Chiller/2(ContactorLine)
  [ProfileBatTemp] -> Chiller/3(ProfileBatTemp)
  ProfBatt_Temp/1 -> [ProfileBatTemp]

== system HIL_Testing_SW/HWO/Charge ==
  Enable : EnablePort  StatesWhenEnabling=reset
  DC : Constant  Value=0  OutDataTypeMode=double  OutDataType=fixdt(1, 16)  OutScaling=2^0  OutDataTypeStr=double
  Period : Constant  Value=0  OutDataTypeMode=double  OutDataType=fixdt(1, 16)  OutScaling=2^0  OutDataTypeStr=double
  Proximity : Constant  Value=0  OutDataTypeMode=boolean  OutDataType=fixdt(1, 16)  OutScaling=2^0  OutDataTypeStr=boolean
  Period_1 : Outport  OutDataType=fixdt(1, 16)  OutScaling=2^0
  DC1 : Outport  Port=2  OutDataType=fixdt(1, 16)  OutScaling=2^0
  Prox : Outport  Port=3  OutDataType=fixdt(1, 16)  OutScaling=2^0
  wires:
  Period/1 -> Period_1/1  "ChargePeriod"
  DC/1 -> DC1/1  "ChargeDC"
  Proximity/1 -> Prox/1  "ChargeProximity"

== system HIL_Testing_SW/HWO/TX HVEM ==
  Current : Inport  OutDataType=sfix(16)  OutScaling=2^0
  CM : Inport  Port=2  OutDataType=sfix(16)  OutScaling=2^0
  Voltage : Inport  Port=3  OutDataType=sfix(16)  OutScaling=2^0
  110V : Constant  OutDataType=fixdt(1, 16)  OutScaling=2^0
  220V : Constant  Value=0  OutDataType=fixdt(1, 16)  OutScaling=2^0
  ChargeCord_Control : Subsystem  AncestorBlock=ChargeCord/ChargeCord_Control  TreatAsAtomicUnit=on
  ChargeCurrent1 : Constant  Value=0  OutDataType=fixdt(1, 16)  OutScaling=2^0
  ChrgCordConnect : Constant  OutDataType=fixdt(1, 16)  OutScaling=2^0
  ChrgCordDisConnect : Constant  Value=0  OutDataType=fixdt(1, 16)  OutScaling=2^0
  Constant : Constant  OutDataType=fixdt(1, 16)  OutScaling=2^0
  Constant1 : Constant  OutDataType=fixdt(1, 16)  OutScaling=2^0
  Divide : Product  Inputs=*/  OutDataType=fixdt(1, 16)  OutScaling=2^-10
  Divide1 : Product  Inputs=*/  OutDataType=fixdt(1, 16)  OutScaling=2^-10
  HVChrgEnStat : Constant  OutDataType=fixdt(1, 16)  OutScaling=2^0
  NoVoltage : Constant  Value=0  OutDataType=fixdt(1, 16)  OutScaling=2^0
  Switch : Switch  Threshold=.5  OutDataType=fixdt(1, 16)  OutScaling=2^0
  Switch1 : Switch  Threshold=.5  OutDataType=fixdt(1, 16)  OutScaling=2^0
  Switch2 : Switch  Threshold=.5  OutDataType=fixdt(1, 16)  OutScaling=2^0  OutDataTypeStr=Inherit: Inherit via back propagation
  Trigger_25ms1 : Subsystem  TreatAsAtomicUnit=on
      settings: CopyFcn=breaklink(gcb)
      mask Type: EnabledFunctionCall
      mask Description:
      | Execute a function-call subsystem at an inherited rate if enabled.
      | 
      | Demux the block's output to execute multiple function-call subsystems in a prescribed order.  The system connected to first demux port is executed first, the system connected to second demux port is executed second, and so on.
      mask Help: web(char(which([char(get_param(gcb,'MaskType')),'.html'])));
      mask Display: disp('f()')
  Voltage1 : Constant  Value=0  OutDataType=fixdt(1, 16)  OutScaling=2^0
  msg_Charge : Subsystem  Tag=x.x
      mask Type: Subsystem
      mask Display:
      | text(.52,.01,char(get_param(gcb,'Tag') ), 'horizontalAlignment','center','verticalAlignment','bottom' )
      | disp(get_param(gcb,'Name'))
  DC : Outport  OutDataType=fixdt(1, 16)  OutScaling=2^0
  Period : Outport  Port=2  OutDataType=fixdt(1, 16)  OutScaling=2^0
  Proximity : Outport  Port=3  OutDataType=fixdt(1, 16)  OutScaling=2^0
  PrcsdVolt_DC : Outport  Port=4  OutDataType=fixdt(1, 16)  OutScaling=2^0
  PrcsdVolt_Period : Outport  Port=5  OutDataType=fixdt(1, 16)  OutScaling=2^0
  wires:
  110V/1 -> ChargeCord_Control/2(110V)
  220V/1 -> ChargeCord_Control/3(220V)
  NoVoltage/1 -> ChargeCord_Control/4(None)
  HVChrgEnStat/1 -> ChargeCord_Control/5(HVChrgACEnStat)
  [voltageChrg] -> msg_Charge/1(HVCD_ACInputVltg)
  [currenChrg] -> msg_Charge/2(HVCD_ACInputCurr)
  [TempChrg] -> msg_Charge/3(HVCD_ACInputTemp)
  ChargeCord_Control/4(Voltage) -> [voltageChrg]
  ChargeCord_Control/5(Current) -> [currenChrg]
  ChargeCord_Control/6(Temp) -> [TempChrg]
  ChargeCurrent1/1 -> Switch/3
  CM/1 -> Switch/2, Switch1/2, Switch2/2
  Current/1 -> Switch/1
  Switch/1 -> msg_Charge/4(Current)
  ChargeCord_Control/2(Ve_OP_t_ControlPilot_ms) -> Divide/2
  Constant/1 -> Divide/1
  ChargeCord_Control/1(Ve_OP_DC_ControlPilot) -> DC/1
  Divide/1 -> Period/1
  ChargeCord_Control/3(Proximity) -> Proximity/1
  Voltage/1 -> Switch1/1
  Voltage1/1 -> Switch1/3
  Switch1/1 -> msg_Charge/5(Voltage)
  ChrgCordConnect/1 -> Switch2/1
  Switch2/1 -> ChargeCord_Control/1(ChrgCordConnect)
  ChrgCordDisConnect/1 -> Switch2/3
  ChargeCord_Control/7(PrcsdVolt_DC) -> PrcsdVolt_DC/1
  Constant1/1 -> Divide1/1
  ChargeCord_Control/8(PrcsdVolt_Freq) -> Divide1/2
  Divide1/1 -> PrcsdVolt_Period/1
  Trigger_25ms1/1(Output Parameter) -> msg_Charge/Trigger

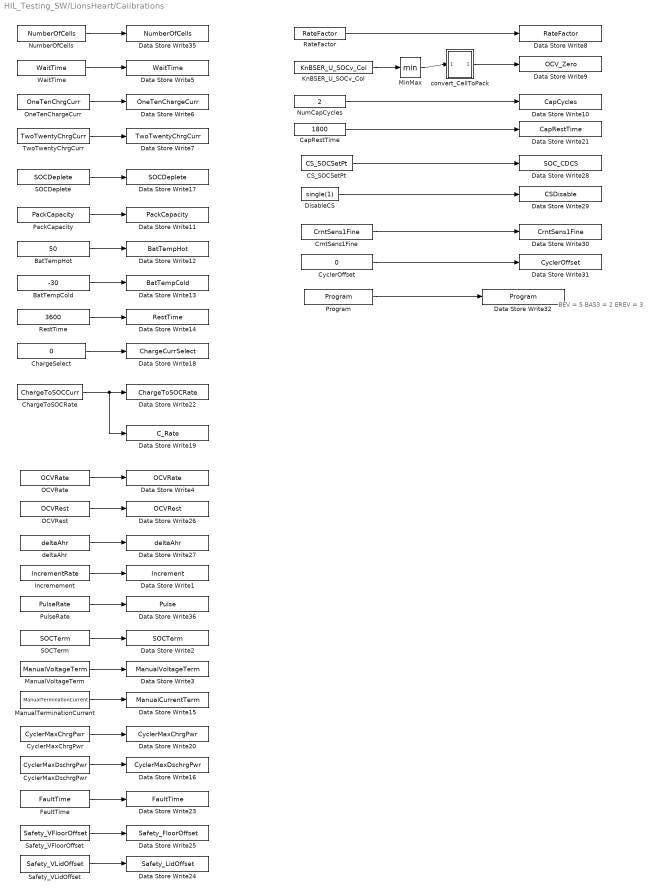
== system HIL_Testing_SW/LionsHeart/Calibrations ==
  note: BEV = 5
      | BAS3 = 2
      | EREV = 3
  BatTempCold : Constant  Value=-30  OutDataTypeMode=single  OutDataType=sfix(16)  OutScaling=2^0  OutDataTypeStr=single
  BatTempHot : Constant  Value=50  OutDataTypeMode=single  OutDataType=sfix(16)  OutScaling=2^0  OutDataTypeStr=single
  CS_SOCSetPt : Constant  Value=CS_SOCSetPt  OutDataType=sfix(16)  OutScaling=2^0
  CapRestTime : Constant  Value=1800  OutDataType=fixdt(1, 16)  OutScaling=2^0  OutDataTypeStr=Inherit: Inherit via back propagation
  ChargeSelect : Constant  Value=0  OutDataType=sfix(16)  OutScaling=2^0
  ChargeToSOCRate : Constant  Value=ChargeToSOCCurr  OutDataTypeMode=single  OutDataType=sfix(16)  OutScaling=2^0  OutDataTypeStr=single
  CrntSens1Fine : Constant  Value=CrntSens1Fine  OutDataType=sfix(16)  OutScaling=2^0
  CyclerMaxChrgPwr : Constant  Value=CyclerMaxChrgPwr  OutDataType=sfix(16)  OutScaling=2^0
  CyclerMaxDschrgPwr : Constant  Value=CyclerMaxDschrgPwr  OutDataType=sfix(16)  OutScaling=2^0
  CyclerOffset : Constant  Value=0  OutDataType=sfix(16)  OutScaling=2^0
  Data Store Write1 : DataStoreWrite  DataStoreName=Increment  SampleTime=-1
  Data Store Write10 : DataStoreWrite  DataStoreName=CapCycles  SampleTime=-1
  Data Store Write11 : DataStoreWrite  DataStoreName=PackCapacity  SampleTime=-1
  Data Store Write12 : DataStoreWrite  DataStoreName=BatTempHot  SampleTime=-1
  Data Store Write13 : DataStoreWrite  DataStoreName=BatTempCold  SampleTime=-1
  Data Store Write14 : DataStoreWrite  DataStoreName=RestTime  SampleTime=-1
  Data Store Write15 : DataStoreWrite  DataStoreName=ManualCurrentTerm  SampleTime=-1
  Data Store Write16 : DataStoreWrite  DataStoreName=CyclerMaxDschrgPwr  SampleTime=-1
  Data Store Write17 : DataStoreWrite  DataStoreName=SOCDeplete  SampleTime=-1
  Data Store Write18 : DataStoreWrite  DataStoreName=ChargeCurrSelect  SampleTime=-1
  Data Store Write19 : DataStoreWrite  DataStoreName=C_Rate  SampleTime=-1
  Data Store Write2 : DataStoreWrite  DataStoreName=SOCTerm  SampleTime=-1
  Data Store Write20 : DataStoreWrite  DataStoreName=CyclerMaxChrgPwr  SampleTime=-1
  Data Store Write21 : DataStoreWrite  DataStoreName=CapRestTime  SampleTime=-1
  Data Store Write22 : DataStoreWrite  DataStoreName=ChargeToSOCRate  SampleTime=-1
  Data Store Write23 : DataStoreWrite  DataStoreName=FaultTime  SampleTime=-1
  Data Store Write24 : DataStoreWrite  DataStoreName=Safety_LidOffset  SampleTime=-1
  Data Store Write25 : DataStoreWrite  DataStoreName=Safety_FloorOffset  SampleTime=-1
  Data Store Write26 : DataStoreWrite  DataStoreName=OCVRest  SampleTime=-1
  Data Store Write27 : DataStoreWrite  DataStoreName=deltaAhr  SampleTime=-1
  Data Store Write28 : DataStoreWrite  DataStoreName=SOC_CDCS  SampleTime=-1
  Data Store Write29 : DataStoreWrite  DataStoreName=CSDisable  SampleTime=-1
  Data Store Write3 : DataStoreWrite  DataStoreName=ManualVoltageTerm  SampleTime=-1
  Data Store Write30 : DataStoreWrite  DataStoreName=CrntSens1Fine  SampleTime=-1
  Data Store Write31 : DataStoreWrite  DataStoreName=CyclerOffset  SampleTime=-1
  Data Store Write32 : DataStoreWrite  DataStoreName=Program  SampleTime=-1
  Data Store Write35 : DataStoreWrite  DataStoreName=NumberOfCells  SampleTime=-1
  Data Store Write36 : DataStoreWrite  DataStoreName=Pulse  SampleTime=-1
  Data Store Write4 : DataStoreWrite  DataStoreName=OCVRate  SampleTime=-1
  Data Store Write5 : DataStoreWrite  DataStoreName=WaitTime  SampleTime=-1
  Data Store Write6 : DataStoreWrite  DataStoreName=OneTenChargeCurr  SampleTime=-1
  Data Store Write7 : DataStoreWrite  DataStoreName=TwoTwentyChrgCurr  SampleTime=-1
  Data Store Write8 : DataStoreWrite  DataStoreName=RateFactor  SampleTime=-1
  Data Store Write9 : DataStoreWrite  DataStoreName=OCV_Zero  SampleTime=-1
  DisableCS : Constant  Value=single(1)  OutDataType=sfix(16)  OutScaling=2^0
  FaultTime : Constant  Value=FaultTime  OutDataType=sfix(16)  OutScaling=2^0
  Incremement : Constant  Value=IncrementRate  OutDataType=sfix(16)  OutScaling=2^0
  KnBSER_U_SOCv_Col : Constant  Value=KnBSER_U_SOCv_Col  OutDataType=fixdt(1, 16)  OutScaling=2^0
  ManualTerminationCurrent : Constant  Value=ManualTerminationCurrent  OutDataType=sfix(16)  OutScaling=2^0
  ManualVoltageTerm : Constant  Value=ManualVoltageTerm  OutDataType=sfix(16)  OutScaling=2^0
  MinMax : MinMax  OutDataType=fixdt(1, 16)  OutScaling=2^0
  NumCapCycles : Constant  Value=2  OutDataType=fixdt(1, 16)  OutScaling=2^0  OutDataTypeStr=Inherit: Inherit via back propagation
  NumberOfCells : Constant  Value=NumberOfCells  OutDataType=sfix(16)  OutScaling=2^0
  OCVRate : Constant  Value=OCVRate  OutDataType=sfix(16)  OutScaling=2^0
  OCVRest : Constant  Value=OCVRest  OutDataType=sfix(16)  OutScaling=2^0
  OneTenChargeCurr : Constant  Value=OneTenChrgCurr  OutDataType=sfix(16)  OutScaling=2^0
  PackCapacity : Constant  Value=PackCapacity  OutDataType=sfix(16)  OutScaling=2^0
  Program : Constant  Value=Program  OutDataTypeMode=double  OutDataType=sfix(16)  OutScaling=2^0  OutDataTypeStr=double
  PulseRate : Constant  Value=PulseRate  OutDataType=sfix(16)  OutScaling=2^0
  RateFactor : Constant  Value=RateFactor  OutDataType=fixdt(1, 16)  OutScaling=2^0
  RestTime : Constant  Value=3600  OutDataTypeMode=single  OutDataType=sfix(16)  OutScaling=2^0  OutDataTypeStr=single
  SOCDeplete : Constant  Value=SOCDeplete  OutDataTypeMode=single  OutDataType=sfix(16)  OutScaling=2^0  OutDataTypeStr=single
  SOCTerm : Constant  Value=SOCTerm  OutDataType=sfix(16)  OutScaling=2^0
  Safety_VFloorOffset : Constant  Value=Safety_VFloorOffset  OutDataType=sfix(16)  OutScaling=2^0
  Safety_VLidOffset : Constant  Value=Safety_VLidOffset  OutDataType=sfix(16)  OutScaling=2^0
  TwoTwentyChrgCurr : Constant  Value=TwoTwentyChrgCurr  OutDataType=sfix(16)  OutScaling=2^0
  WaitTime : Constant  Value=WaitTime  OutDataType=sfix(16)  OutScaling=2^0
  convert_CellToPack : Subsystem
  deltaAhr : Constant  Value=deltaAhr  OutDataType=sfix(16)  OutScaling=2^0
  wires:
  NumberOfCells/1 -> Data Store Write35/1
  WaitTime/1 -> Data Store Write5/1
  OneTenChargeCurr/1 -> Data Store Write6/1
  TwoTwentyChrgCurr/1 -> Data Store Write7/1
  PackCapacity/1 -> Data Store Write11/1
  BatTempHot/1 -> Data Store Write12/1
  BatTempCold/1 -> Data Store Write13/1
  RestTime/1 -> Data Store Write14/1
  ChargeSelect/1 -> Data Store Write18/1
  SOCDeplete/1 -> Data Store Write17/1
  OCVRate/1 -> Data Store Write4/1
  OCVRest/1 -> Data Store Write26/1
  deltaAhr/1 -> Data Store Write27/1
  Incremement/1 -> Data Store Write1/1
  PulseRate/1 -> Data Store Write36/1
  ChargeToSOCRate/1 -> Data Store Write22/1, Data Store Write19/1
  SOCTerm/1 -> Data Store Write2/1
  ManualVoltageTerm/1 -> Data Store Write3/1
  ManualTerminationCurrent/1 -> Data Store Write15/1
  CyclerMaxChrgPwr/1 -> Data Store Write20/1
  CyclerMaxDschrgPwr/1 -> Data Store Write16/1
  FaultTime/1 -> Data Store Write23/1
  Safety_VFloorOffset/1 -> Data Store Write25/1
  Safety_VLidOffset/1 -> Data Store Write24/1
  RateFactor/1 -> Data Store Write8/1
  KnBSER_U_SOCv_Col/1 -> MinMax/1
  MinMax/1 -> convert_CellToPack/1(In1)
  convert_CellToPack/1(Out1) -> Data Store Write9/1
  NumCapCycles/1 -> Data Store Write10/1
  CapRestTime/1 -> Data Store Write21/1
  CS_SOCSetPt/1 -> Data Store Write28/1
  DisableCS/1 -> Data Store Write29/1
  CrntSens1Fine/1 -> Data Store Write30/1
  CyclerOffset/1 -> Data Store Write31/1
  Program/1 -> Data Store Write32/1
